simulink model "testPIArduino"  (R2013a)
settings: Solver=ode3  SolverMode=SingleTasking  StartTime=0.0  StopTime=inf  FixedStep=0.1  RelTol=1e-3
model workspace (MAT data in the model file):
  blc = -50
  brc = -50
  flc = 50
  frc = 50
  rc = 0
libraries: arduinolib x4, simulink x3, dspbuff3 x1
settings Model: SimulationMode=external  ExtModeTrigDuration=100  Creator=sbiagion  LastModifiedBy=scastro
settings DataIOCC: SignalLoggingSaveFormat=ModelDataLogs
settings OptimizationCC: OptimizeModelRefInitCode=on  LifeSpan=1
settings DebuggingCC: SolverPrmCheckMsg=none  MultiTaskDSMMsg=warning  MultiTaskCondExecSysMsg=none  StateNameClashWarn=none  StrictBusMsg=None
settings HardwareCC: ProdBitPerInt=16  ProdBitPerPointer=8  ProdIntDivRoundTo=Zero  ProdEndianess=LittleEndian  ProdWordSize=8  ProdHWDeviceType=Atmel->AVR
settings RTWCC: SystemTargetFile=realtime.tlc  GenerateMakefile=off  TemplateMakefile=realtime.tmf  Description=Run on Target Hardware  RTWVerbose=off  ProcessScript=realtime_make_rtw_hook  IncludeERTFirstTime=on
settings STFCustomTargetCC: TargetLibSuffix=.a  GenerateSampleERTMain=on  ERTCustomFileBanners=on  SupportNonInlinedSFcns=off  SupportVariableSizeSignals=on  MATLABClassNameForMDSCustomization=Simulink.SoftwareTarget.ERTCustomization  SystemTargetFile=realtime.tlc
settings ERTTargetCC: ParMdlRefBuildCompliant=off  CompOptLevelCompliant=off  ConcurrentExecutionCompliant=off  CombineOutputUpdateFcns=off  ERTFirstTimeCompliant=off  SupportContinuousTime=on  SupportVariableSizeSignals=on  ModelStepFunctionPrototypeControlCompliant=off  CPPClassGenCompliant=off  ExtMode=on  ExtModeTransport=3  ExtModeMexFile=ext_serial_win32_comm  ExtModeMexArgs=0 52 115200  ERTSrcFileBannerTemplate=realtime_code_template.cgt  ERTHdrFileBannerTemplate=realtime_code_template.cgt  ERTDataSrcFileTemplate=realtime_code_template.cgt  ERTDataHdrFileTemplate=realtime_code_template.cgt  ERTCustomFileTemplate=realtime_file_process.tlc

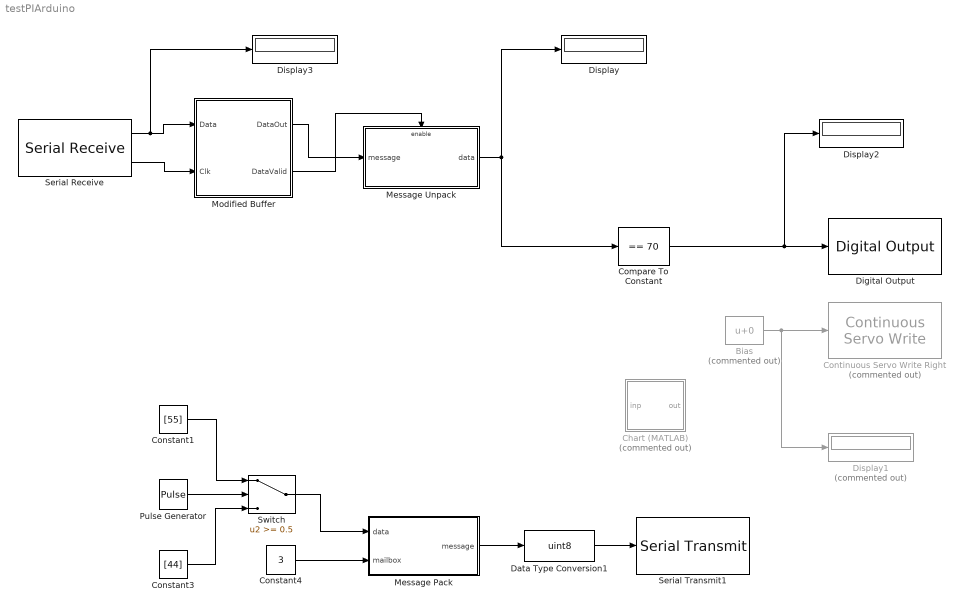
== system testPIArduino ==
  Bias : Bias  Commented=on
  Chart (MATLAB) : Stateflow chart  Commented=on  TreatAsAtomicUnit=on
  Compare To Constant : simulink/Logic and Bit Operations/Compare To Constant  relop===  const=70  OutDataTypeStr=boolean
  Constant1 : Constant  Value=[55]
  Constant3 : Constant  Value=[44]
  Constant4 : Constant  Value=3
  Continuous Servo Write Right : arduinolib/Continuous Servo Write  Commented=on  pinNumber=49
  Data Type Conversion1 : DataTypeConversion  OutDataTypeStr=uint8
  Digital Output : arduinolib/Digital Output  pinNumber=13
  Display : Display
  Display1 : Display  Commented=on
  Display2 : Display
  Display3 : Display
  Message Pack : Subsystem
  Message Unpack : Subsystem  TreatAsAtomicUnit=on
  Modified Buffer : Subsystem  TreatAsAtomicUnit=on  mask(Input-Driven Buffer){bufSize=4}
      mask prompts: bufSize "Buffer size:"
      mask help: A modified buffer subsystem that is driven by the arrival of its input data; it produces a valid output data buffer whenever its buffer is full and sets its dataValid flag to 1. Otherwise, the data at its dataOut port is not valid and its dataValid flag is set to 0.
      settings: AttributesFormatString=Counting Buffer
      mask Display: disp('Modified Buffer')
  Pulse Generator : DiscretePulseGenerator  PulseType=Time based  Period=4  PulseWidth=50
  Serial Receive : arduinolib/Serial Receive  portNumber=1  showOutStatus=on  sampleTime=0.1
  Serial Transmit1 : arduinolib/Serial Transmit  portNumber=1
  Switch : Switch  Threshold=0.5
  wires:
  Bias/1 -> Display1/1, Continuous Servo Write Right/1
  Compare To Constant/1 -> Display2/1, Digital Output/1
  Message Unpack/1(data) -> Compare To Constant/1, Display/1
  Serial Receive/1 -> Display3/1, Modified Buffer/1(Data)
  Serial Receive/2 -> Modified Buffer/2(Clk)
  Modified Buffer/2(DataValid) -> Message Unpack/Enable
  Modified Buffer/1(DataOut) -> Message Unpack/1(message)
  Constant4/1 -> Message Pack/2(mailbox)
  Message Pack/1(message) -> Data Type Conversion1/1
  Constant1/1 -> Switch/1
  Constant3/1 -> Switch/3
  Pulse Generator/1 -> Switch/2
  Data Type Conversion1/1 -> Serial Transmit1/1
  Switch/1 -> Message Pack/1(data)

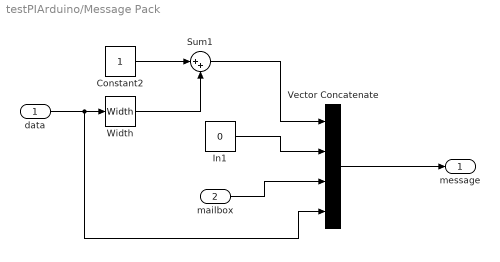
== system testPIArduino/Message Pack ==
  data : Inport
  mailbox : Inport  Port=2
  Constant2 : Constant
  In1 : Constant  Value=0
  Sum1 : Sum  Inputs=|++
  Vector Concatenate : Concatenate  NumInputs=4
  Width : Width
  message : Outport
  wires:
  Constant2/1 -> Sum1/1
  In1/1 -> Vector Concatenate/2
  data/1 -> Vector Concatenate/4, Width/1
  Vector Concatenate/1 -> message/1
  mailbox/1 -> Vector Concatenate/3
  Sum1/1 -> Vector Concatenate/1
  Width/1 -> Sum1/2

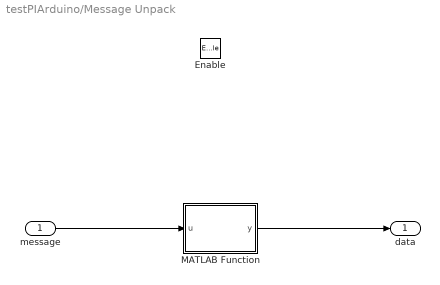
== system testPIArduino/Message Unpack ==
  message : Inport
  Enable : EnablePort
  MATLAB Function : MATLAB Function  TreatAsAtomicUnit=on
  data : Outport
  wires:
  message/1 -> MATLAB Function/1(u)
  MATLAB Function/1(y) -> data/1

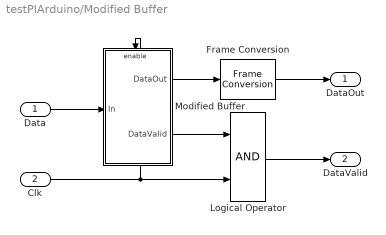
== system testPIArduino/Modified Buffer ==
  Data : Inport
  Clk : Inport  Port=2
  Frame Conversion : FrameConversion  OutFrame=Sample-based
  Logical Operator : Logic  AllPortsSameDT=off  OutDataTypeStr=boolean
  Modified Buffer : Subsystem
  DataOut : Outport
  DataValid : Outport  Port=2
  wires:
  Clk/1 -> Logical Operator/2, Modified Buffer/Enable
  Frame Conversion/1 -> DataOut/1
  Logical Operator/1 -> DataValid/1
  Modified Buffer/2(DataValid) -> Logical Operator/1
  Modified Buffer/1(DataOut) -> Frame Conversion/1
  Data/1 -> Modified Buffer/1(In)

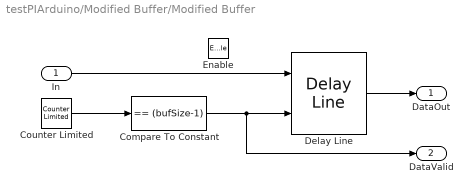
== system testPIArduino/Modified Buffer/Modified Buffer ==
  In : Inport
  Enable : EnablePort
  Compare To Constant : simulink/Logic and Bit Operations/Compare To Constant  relop===  const=(bufSize-1)  OutDataTypeStr=boolean  ZeroCross=off
  Counter Limited : simulink/Sources/Counter Limited  uplimit=(bufSize-1)  tsamp=-1
  Delay Line : dspbuff3/Delay Line  siz=bufSize  ic=0  directfeed=on  enable_output=on  hold_output=off  TreatMby1Signals=One channel
  DataOut : Outport
  DataValid : Outport  Port=2
  wires:
  Counter Limited/1 -> Compare To Constant/1
  In/1 -> Delay Line/1
  Delay Line/1 -> DataOut/1
  Compare To Constant/1 -> DataValid/1, Delay Line/2

== matlab function testPIArduino/Message Unpack/MATLAB Function ==
  data: u input; y output
function y = fcn(u)
%#codegen

zero_index = find(u==0);
if zero_index(1)+2<=4
    value_index = zero_index(1)+2;
else
    value_index = mod((zero_index(1)+2),4);
end
y = u(value_index);

== stateflow chart testPIArduino/Chart (MATLAB) ==
  (default) -> (junction 2) : {out = isequal(inp,StatusID.YOSHI_SENSED_RAMP);}
  data: out output; inp input
